simulink model "dirdyna_CoMan_23Dof_V4"  (Simulink 8.1)
settings: Solver=ode4  StartTime=0  StopTime=30  FixedStep=0.0005  MaxStep=1e-2  RelTol=1e-3  AbsTol=1e-6
undefined symbols (not defined in the file or in its folder): Function_dirdynared, MBStoAnimFile_StopFcnCallback, Modules, Robotran, S
settings Model: Creator=nvandernoot  LastModifiedBy=nvandernoot
settings SolverCC: InitialStep=1e-3

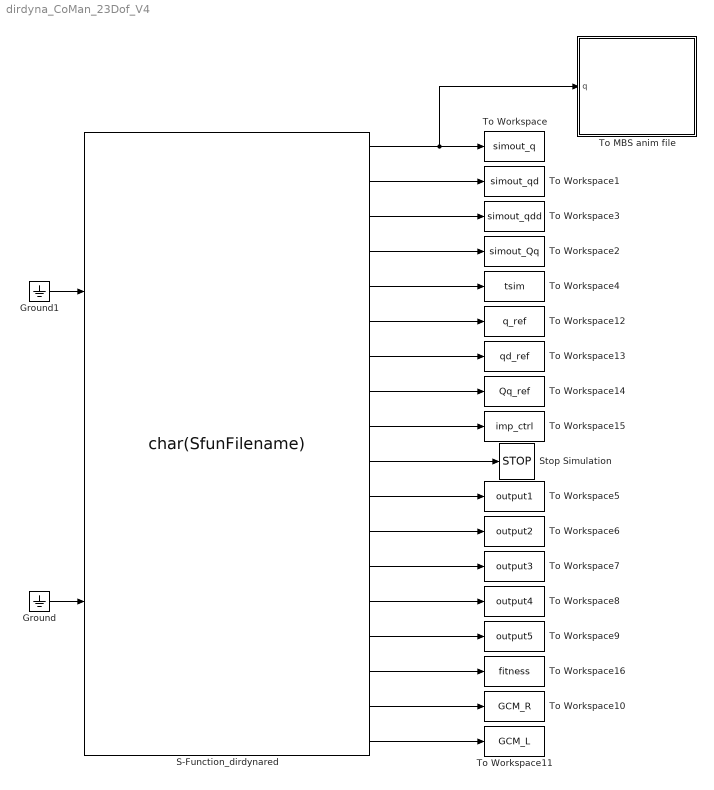
== system dirdyna_CoMan_23Dof_V4 ==
  Ground : Ground
  Ground1 : Ground
  S-Function_dirdynared : S-Function  AncestorBlock=Robotran/Modules/S-Function_dirdynared  FunctionName=char(SfunFilename)  Parameters=getfield(get(gcbh,'UserData'),'mbs_data') q_ini  EnableBusSupport=off  mask(S-function: Robotran Direct Dynamics (dirdynared)){SfunFilename=mbs_sf_dirdynared_CoMan_23Dof_V4, q_ini=off, creation_date=29-Oct-2013}
      mask prompts: SfunFilename "S-function filename"; q_ini "Get initial qu from block inputs"; creation_date "Enter the creation date:"
      mask help: Compute the Direct Dynamics equations using symbolic MBS formalism
      settings: OpenFcn=MBSdirdynaredSfunction
      settings: CopyFcn=|
      | MBSdirdynaredSfunction;
      | set_param(gcs,'MaxStep','1e-2');
      | set_param(gcs,'InitialStep','1e-3');
      | set_param(gcs,'RelTol','1e-3');
      | set_param(gcs,'AbsTol','1e-6');
      | set_param(gcb,'OpenFcn','MBSdirdynaredSfunction');
      | set_param(gcb,'creation_date',date);
      mask Display:
      | disp('Robotran\nDirect\nDynamics\n(dirdynared)\n-\n CoMan_23Dof_V4\n-\n29-Oct-2013');
      | port_label('input',1,'Joint forces');
      | port_label('input',2,'Driven joints');
      | port_label('output',1,'q');
      | port_label('output',2,'qd');
      | port_label('output',3,'qdd');
  Stop Simulation : Stop
  To MBS anim file : Subsystem  AncestorBlock=Robotran/Utilities/To MBS anim file  StopFcn=MBStoAnimFile_StopFcnCallback;  mask{varname=tqres, filename=simdir.anim, prjname=CoMan_23Dof_V4, overwrite=0, samplingRate=1000}
      mask prompts: varname "variable name"; filename "anim file name"; prjname "project name"; samplingRate "sampling rate"
      settings: CopyFcn=MBStoAnimFile_v2;  OpenFcn=MBStoAnimFile_v2;
      mask Display: image(imread('Logo_anim.jpg'))
  To Workspace : ToWorkspace  VariableName=simout_q  SampleTime=-1  SaveFormat=Structure
  To Workspace1 : ToWorkspace  VariableName=simout_qd  SampleTime=-1  SaveFormat=Structure
  To Workspace10 : ToWorkspace  VariableName=GCM_R  SampleTime=-1  SaveFormat=Structure
  To Workspace11 : ToWorkspace  VariableName=GCM_L  SampleTime=-1  SaveFormat=Structure
  To Workspace12 : ToWorkspace  VariableName=q_ref  SampleTime=-1  SaveFormat=Structure
  To Workspace13 : ToWorkspace  VariableName=qd_ref  SampleTime=-1  SaveFormat=Structure
  To Workspace14 : ToWorkspace  VariableName=Qq_ref  SampleTime=-1  SaveFormat=Structure
  To Workspace15 : ToWorkspace  VariableName=imp_ctrl  SampleTime=-1  SaveFormat=Structure
  To Workspace16 : ToWorkspace  VariableName=fitness  SampleTime=-1  SaveFormat=Structure
  To Workspace2 : ToWorkspace  VariableName=simout_Qq  SampleTime=-1  SaveFormat=Structure
  To Workspace3 : ToWorkspace  VariableName=simout_qdd  SampleTime=-1  SaveFormat=Structure
  To Workspace4 : ToWorkspace  VariableName=tsim  SampleTime=-1  SaveFormat=Structure
  To Workspace5 : ToWorkspace  VariableName=output1  SampleTime=-1  SaveFormat=Structure
  To Workspace6 : ToWorkspace  VariableName=output2  SampleTime=-1  SaveFormat=Structure
  To Workspace7 : ToWorkspace  VariableName=output3  SampleTime=-1  SaveFormat=Structure
  To Workspace8 : ToWorkspace  VariableName=output4  SampleTime=-1  SaveFormat=Structure
  To Workspace9 : ToWorkspace  VariableName=output5  SampleTime=-1  SaveFormat=Structure
  wires:
  Ground1/1 -> S-Function_dirdynared/1
  Ground/1 -> S-Function_dirdynared/2
  S-Function_dirdynared/1 -> To Workspace/1, To MBS anim file/1(q)
  S-Function_dirdynared/2 -> To Workspace1/1
  S-Function_dirdynared/3 -> To Workspace3/1
  S-Function_dirdynared/4 -> To Workspace2/1
  S-Function_dirdynared/5 -> To Workspace4/1
  S-Function_dirdynared/6 -> To Workspace12/1
  S-Function_dirdynared/7 -> To Workspace13/1
  S-Function_dirdynared/8 -> To Workspace14/1
  S-Function_dirdynared/9 -> To Workspace15/1
  S-Function_dirdynared/10 -> Stop Simulation/1
  S-Function_dirdynared/11 -> To Workspace5/1
  S-Function_dirdynared/12 -> To Workspace6/1
  S-Function_dirdynared/13 -> To Workspace7/1
  S-Function_dirdynared/14 -> To Workspace8/1
  S-Function_dirdynared/15 -> To Workspace9/1
  S-Function_dirdynared/16 -> To Workspace16/1
  S-Function_dirdynared/17 -> To Workspace10/1
  S-Function_dirdynared/18 -> To Workspace11/1

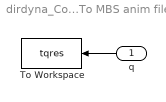
== system dirdyna_CoMan_23Dof_V4/To MBS anim file ==
  q : Inport
  To Workspace : ToWorkspace  VariableName=tqres  SampleTime=-1  SaveFormat=Structure With Time
  wires:
  q/1 -> To Workspace/1
